simulink model "NN_Blackbox_comparison_Sinusoidal_24_24_6"  (R2019a)
settings: Solver=FixedStepAuto  StartTime=0.0  StopTime=10  FixedStep=0.01  RelTol=1e-3
undefined symbols (not defined in the file or in its folder): B, b, l, m, R
libraries: neural x17
(part 2 of 2)

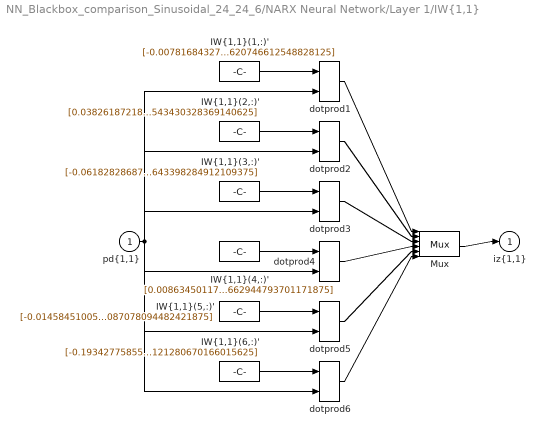
== system NN_Blackbox_comparison_Sinusoidal_24_24_6/NARX Neural Network/Layer 1/IW{1,1} ==
  "pd{1,1}" : Inport  PortDimensions=24  SampleTime=0.01
      mask Display: e = 0.06;c1 = [120 230 180]/255;c2 = ([120 230 180]+0)/(256+128);c3 = ([120 230 180]+128)/(256+128);patch([0 1 1 0],[0 0 1 1],c1);patch([0 1 1 1-e 1-e 0+e],[0 0 1 1-e 0+e 0+e],c2);patch([0 0 1 1-e 0+e 0+e],[0 1 1 1-e 1-e 0+e],c3);plot([0 1 1 0 0],[0 0 1 1 0]);
  "IW{1,1}(1,:)'" : Constant  Value=[-0.00781684327807324365322561021685032756067812442779541015625;-0.1850159880792916766711897480490733869373798370361328125;0.1001605115023758985071111737852334044873714447021484375;-0.1833831276225645068311820296003133989870548248291015625;-0.0494952264880428038917870026125456206500530242919921875;-0.0199884323316934509051634449861012399196624755859375;0.1165778684201735082570650092748110182583332061767578125;-0.1146125589407599176805518936816952191293239593505859375;0.05020117748370077348507578562930575571954250335693359375;-0.07054520144965477357335004171545733697712421417236328125;0.06259819221112832010600612875350634567439556121826171875;0.1424776467193929196941581949431565590202808380126953125;-0.133745237374407854868962886030203662812709808349609375;0.0296684098027802482799852867856316152028739452362060546875;0.00161749987780685660666846192867751597077585756778717041015625;-0.082135310527604088459696640711626969277858734130859375;0.017117640879136607201527198185431188903748989105224609375;-0.06257214896964193029393896949841291643679141998291015625;0.044772057090533036449730985850692377425730228424072265625;0.077435295268282799963088791628251783549785614013671875;0.05627579238971676389713394428326864726841449737548828125;-0.021855753086099154181010106867688591592013835906982421875;-0.1460877193397679130182353901545866392552852630615234375;-0.03835883480631437081331824856533785350620746612548828125]
      mask Display: e = 0.06;c1 = [120 150 230]/255;c2 = ([120 150 230]+0)/383;c3 = ([120 150 230]+128)/383;patch([0 1 1 0],[0 0 1 1],c1);patch([0 1 1 1-e 1-e 0+e],[0 0 1 1-e 0+e 0+e],c2);patch([0 0 1 1-e 0+e 0+e],[0 1 1 1-e 1-e 0+e],c3);plot([0 1 1 0 0],[0 0 1 1 0]);disp('Weights');
  "IW{1,1}(2,:)'" : Constant  Value=[0.0382618721846479659109974136299570091068744659423828125;-0.11423689285097904377863642366719432175159454345703125;0.133546945696815633208842655221815221011638641357421875;0.1881509242216309052420086800339049659669399261474609375;-0.310690738266952648505281331381411291658878326416015625;0.08079194265866813939869217620071140117943286895751953125;-0.1261531193252228566503703177659190259873867034912109375;0.22552293164817882598072174005210399627685546875;-0.262279279918452068454115533313597552478313446044921875;0.07233767871772382729300687742579611949622631072998046875;-0.0205932665107694153061590469633301836438477039337158203125;-0.1546453563928802121818506520867231301963329315185546875;0.036264331257236916139508053902318351902067661285400390625;0.04911111148654201397079077651142142713069915771484375;-0.13793151140202575266613393978332169353961944580078125;-0.07579443180956568770767489695572294294834136962890625;0.09929461869162765907947942878308822400867938995361328125;0.132426095028207180259727238080813549458980560302734375;-0.221957074010017019194407339455210603773593902587890625;-0.348947713802484626999245165279717184603214263916015625;-0.06397706287970154892530416645968216471374034881591796875;-0.08647843787593545439307263222872279584407806396484375;0.17868669570401685131599833766813389956951141357421875;0.1398750507253951058661556317019858397543430328369140625]
      mask Display: e = 0.06;c1 = [120 150 230]/255;c2 = ([120 150 230]+0)/383;c3 = ([120 150 230]+128)/383;patch([0 1 1 0],[0 0 1 1],c1);patch([0 1 1 1-e 1-e 0+e],[0 0 1 1-e 0+e 0+e],c2);patch([0 0 1 1-e 0+e 0+e],[0 1 1 1-e 1-e 0+e],c3);plot([0 1 1 0 0],[0 0 1 1 0]);disp('Weights');
  "IW{1,1}(3,:)'" : Constant  Value=[-0.061828286876414721706662902533935266546905040740966796875;-0.188069077398500261733005345377023331820964813232421875;-0.05601321185507872335573864575053448788821697235107421875;-0.855195451738412604214545353897847235202789306640625;-0.02152969126247221420822341997336479835212230682373046875;-0.1226276060420865288147496130477520637214183807373046875;0.54597989168019134265108505132957361638545989990234375;-0.472796354773704685658941571091418154537677764892578125;-0.05967068096914411590159232900987262837588787078857421875;0.07449502355572552858564705502431024797260761260986328125;0.432613897270532843375434595145634375512599945068359375;0.62244785617741282823800474943709559738636016845703125;-0.40187421715495552643204746345872990787029266357421875;0.11617911031940737764944771015507285483181476593017578125;-0.027881334145780554967242181874098605476319789886474609375;-0.2104685385077245118878863650024868547916412353515625;-0.0772998380072060786716292568598873913288116455078125;-0.37592925407182342656398077451740391552448272705078125;0.41876994636821718298591576967737637460231781005859375;0.63252910097631287467123684109537862241268157958984375;-0.07433228516414784603494325665451469831168651580810546875;0.01353334729246670649349670867422901210375130176544189453125;-0.62092193287436103776855134128709323704242706298828125;-0.486445315902774344518633142797625623643398284912109375]
      mask Display: e = 0.06;c1 = [120 150 230]/255;c2 = ([120 150 230]+0)/383;c3 = ([120 150 230]+128)/383;patch([0 1 1 0],[0 0 1 1],c1);patch([0 1 1 1-e 1-e 0+e],[0 0 1 1-e 0+e 0+e],c2);patch([0 0 1 1-e 0+e 0+e],[0 1 1 1-e 1-e 0+e],c3);plot([0 1 1 0 0],[0 0 1 1 0]);disp('Weights');
  "IW{1,1}(4,:)'" : Constant  Value=[0.00863450117239293428450519485295444610528647899627685546875;-0.000724270040755028749086819050972962941159494221210479736328125;0.0037910992940890044823609716928558555082418024539947509765625;0.00121298856381454205934089518592600143165327608585357666015625;0.0021858889202538661460095692490313012967817485332489013671875;0.0015493290437253895257263547335924158687703311443328857421875;0.00138676077665267328230258581100997616886161267757415771484375;0.00116498878916462887504745804534422859433107078075408935546875;0.000675385155924593358518770447318502192501910030841827392578125;0.000216059403336755378489952850173949627787806093692779541015625;0.000561817516077093973871081633575386149459518492221832275390625;0.000502256192877557319960424297988765829359181225299835205078125;0.0004713245037647317684827152906024139156215824186801910400390625;0.000252772431095591256812460390079877470270730555057525634765625;-9.378217509820683931744123018603431773954071104526519775390625e-05;-9.917273133467054894822634292239627029630355536937713623046875e-05;0.00022807121218579545600391167425868843565694987773895263671875;6.01539461235079875507138214008051591008552350103855133056640625e-05;0.00050922601514351360611765340280499003711156547069549560546875;-0.0003978415441667664041551499831683713637175969779491424560546875;0.00048009319238550250685815257156718871556222438812255859375;-0.0003596580952784336391268860122494288589223287999629974365234375;-7.3598210936802051468190455363327373561332933604717254638671875e-05;-0.00022865933921139785611580108604101724267820827662944793701171875]
      mask Display: e = 0.06;c1 = [120 150 230]/255;c2 = ([120 150 230]+0)/383;c3 = ([120 150 230]+128)/383;patch([0 1 1 0],[0 0 1 1],c1);patch([0 1 1 1-e 1-e 0+e],[0 0 1 1-e 0+e 0+e],c2);patch([0 0 1 1-e 0+e 0+e],[0 1 1 1-e 1-e 0+e],c3);plot([0 1 1 0 0],[0 0 1 1 0]);disp('Weights');
  "IW{1,1}(5,:)'" : Constant  Value=[-0.01458451005635619072975384113988184253685176372528076171875;-6.42425160279898690464384092280170079902745783329010009765625e-05;0.000617139824523241513516691458818286264431662857532501220703125;-0.0004628604352088678554853762303622488616383634507656097412109375;0.0002626759407408229434789659340054868152947165071964263916015625;0.00010283267385660473298460149127464546836563386023044586181640625;-0.00075071973850503507207088116359727791859768331050872802734375;0.0007176821664602243792951963285986494156531989574432373046875;-0.001986327739272509933232679912862295168451964855194091796875;-0.001627764366681831893768350738582739722914993762969970703125;-0.0004169956863333358957311725045968842096044681966304779052734375;-0.0018908506049463806586441450008351239375770092010498046875;9.8008331296605655474744878130621827949653379619121551513671875e-05;-0.0013958936559834863276596816916708121425472199916839599609375;-0.0022485379598983609890361368144340303842909634113311767578125;-0.00108820154986972463494188101407189606106840074062347412109375;-0.00049658626834902315667907846119533132878132164478302001953125;-0.0009511741998911474142708311063643122906796634197235107421875;0.0003314857832199900725990426852973769200616516172885894775390625;-0.003139569163090162075280264986076872446574270725250244140625;-0.00017847932028995896667177001315707229878171347081661224365234375;-0.002218879578591786451424727744097253889776766300201416015625;-0.000318328681633440655450451028940506148501299321651458740234375;-0.00113966174305159153971878094324665653402917087078094482421875]
      mask Display: e = 0.06;c1 = [120 150 230]/255;c2 = ([120 150 230]+0)/383;c3 = ([120 150 230]+128)/383;patch([0 1 1 0],[0 0 1 1],c1);patch([0 1 1 1-e 1-e 0+e],[0 0 1 1-e 0+e 0+e],c2);patch([0 0 1 1-e 0+e 0+e],[0 1 1 1-e 1-e 0+e],c3);plot([0 1 1 0 0],[0 0 1 1 0]);disp('Weights');
  "IW{1,1}(6,:)'" : Constant  Value=[-0.19342775855704219534203502917080186307430267333984375;0.1533401124560897776927248514766688458621501922607421875;-0.465714971164614188747776779564446769654750823974609375;-0.2452381847837121764399626044905744493007659912109375;-0.437933644939707600318712366060935892164707183837890625;0.0224203308941918477703580947490991093218326568603515625;0.6222688006434211605011341816862113773822784423828125;0.54116406477055345458637702904525212943553924560546875;0.55228269096517623726327883559861220419406890869140625;-0.364776363386681234945996266105794347822666168212890625;0.5125049224945821269017187660210765898227691650390625;-0.3208727112808242853958518026047386229038238525390625;0.26590788638917650654747149019385688006877899169921875;-0.42450676756308725057209585429518483579158782958984375;0.06490358610860956500854257456012419424951076507568359375;0.0253195955065332427291746597575183841399848461151123046875;0.1263078999877178254518383937465841881930828094482421875;-0.41212086410198878194677263309131376445293426513671875;-0.0396676510640926738293643438737490214407444000244140625;0.374919128482076313702009429107420146465301513671875;-0.262882740181810070634327303196187131106853485107421875;-0.420155000962919966678299488194170407950878143310546875;-0.682896272804139670142831164412200450897216796875;-0.031254028514375566116800797544783563353121280670166015625]
      mask Display: e = 0.06;c1 = [120 150 230]/255;c2 = ([120 150 230]+0)/383;c3 = ([120 150 230]+128)/383;patch([0 1 1 0],[0 0 1 1],c1);patch([0 1 1 1-e 1-e 0+e],[0 0 1 1-e 0+e 0+e],c2);patch([0 0 1 1-e 0+e 0+e],[0 1 1 1-e 1-e 0+e],c3);plot([0 1 1 0 0],[0 0 1 1 0]);disp('Weights');
  Mux : Mux  Inputs=6
      mask Display: e = 0.06;c1 = [120 150 230]/255;c2 = ([120 150 230]+0)/383;c3 = ([120 150 230]+128)/383;patch([0 1 1 0],[0 0 1 1],c1);patch([0 1 1 1-e 1-e 0+e],[0 0 1 1-e 0+e 0+e],c2);patch([0 0 1 1-e 0+e 0+e],[0 1 1 1-e 1-e 0+e],c3);plot([0 1 1 0 0],[0 0 1 1 0]);disp('Mux');
  dotprod{1..6} (6 alike) : neural/Weight Functions/dotprod
      settings: SourceProductName=MATLAB Runtime - Deep Learning Toolbox  SourceProductBaseCode=Missing
  "iz{1,1}" : Outport
      mask Display: e = 0.06;c1 = [120 230 180]/255;c2 = ([120 230 180]+0)/(256+128);c3 = ([120 230 180]+128)/(256+128);patch([0 1 1 0],[0 0 1 1],c1);patch([0 1 1 1-e 1-e 0+e],[0 0 1 1-e 0+e 0+e],c2);patch([0 0 1 1-e 0+e 0+e],[0 1 1 1-e 1-e 0+e],c3);plot([0 1 1 0 0],[0 0 1 1 0]);
  wires:
  "IW{1,1}(1,:)'"/1 -> dotprod1/1
  "pd{1,1}"/1 -> dotprod1/2, dotprod2/2, dotprod3/2, dotprod4/2, dotprod5/2, dotprod6/2
  dotprod1/1 -> Mux/1
  "IW{1,1}(2,:)'"/1 -> dotprod2/1
  dotprod2/1 -> Mux/2
  "IW{1,1}(3,:)'"/1 -> dotprod3/1
  dotprod3/1 -> Mux/3
  "IW{1,1}(4,:)'"/1 -> dotprod4/1
  dotprod4/1 -> Mux/4
  "IW{1,1}(5,:)'"/1 -> dotprod5/1
  dotprod5/1 -> Mux/5
  "IW{1,1}(6,:)'"/1 -> dotprod6/1
  dotprod6/1 -> Mux/6
  Mux/1 -> "iz{1,1}"/1

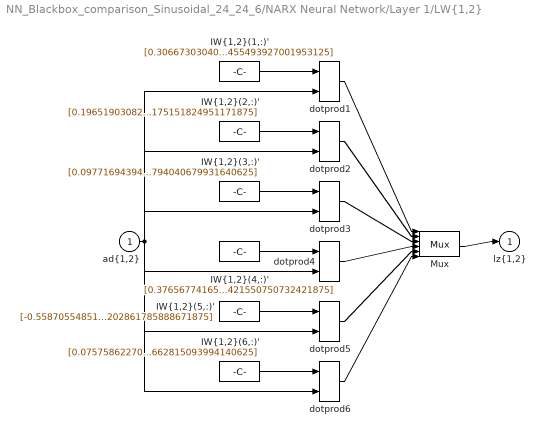
== system NN_Blackbox_comparison_Sinusoidal_24_24_6/NARX Neural Network/Layer 1/LW{1,2} ==
  "ad{1,2}" : Inport  PortDimensions=24  SampleTime=0.01
      mask Display: e = 0.06;c1 = [120 230 180]/255;c2 = ([120 230 180]+0)/(256+128);c3 = ([120 230 180]+128)/(256+128);patch([0 1 1 0],[0 0 1 1],c1);patch([0 1 1 1-e 1-e 0+e],[0 0 1 1-e 0+e 0+e],c2);patch([0 0 1 1-e 0+e 0+e],[0 1 1 1-e 1-e 0+e],c3);plot([0 1 1 0 0],[0 0 1 1 0]);
  "IW{1,2}(1,:)'" : Constant  Value=[0.306673030408703917171209241132601164281368255615234375;-0.11198177206757127521985495377521147020161151885986328125;0.3269859355907691611520249352906830608844757080078125;0.056270185849424024515652575928470469079911708831787109375;-0.113558622384051233211721410043537616729736328125;0.09782792362847221590005375446708058007061481475830078125;-0.3122359510233196910888864294975064694881439208984375;-0.257081540505827488285461868144921027123928070068359375;0.276391847125739553714396379291429184377193450927734375;0.2222602218884729696757318606614717282354831695556640625;-0.2021395968177663593490223092885571531951427459716796875;0.1814053757736827365842913195592700503766536712646484375;0.2258593327786559690206757977648521773517131805419921875;-0.2029117090672250822702693540122709237039089202880859375;0.0282557608137135353454372221904122852720320224761962890625;-0.230249871903323855004686038228101097047328948974609375;-0.2195438158585874266481852146171149797737598419189453125;0.261170925858878799630247158347629010677337646484375;0.180486427927954939942623013848788104951381683349609375;0.069226347620993278209056143168709240853786468505859375;-0.1443199707426636724250101906363852322101593017578125;-0.2391833789258829556789720527376630343496799468994140625;0.1659067472852251701187498156286892481148242950439453125;0.11194979810412608589587080132332630455493927001953125]
      mask Display: e = 0.06;c1 = [120 150 230]/255;c2 = ([120 150 230]+0)/383;c3 = ([120 150 230]+128)/383;patch([0 1 1 0],[0 0 1 1],c1);patch([0 1 1 1-e 1-e 0+e],[0 0 1 1-e 0+e 0+e],c2);patch([0 0 1 1-e 0+e 0+e],[0 1 1 1-e 1-e 0+e],c3);plot([0 1 1 0 0],[0 0 1 1 0]);disp('weights');
  "IW{1,2}(2,:)'" : Constant  Value=[0.196519030828230689689206656112219206988811492919921875;-0.1595862747555963634393805250510922633111476898193359375;-0.238312071756647425591069122674525715410709381103515625;-0.37667022763899893345040936765144579112529754638671875;-0.01219480248024964845476869612639347906224429607391357421875;-0.16186153809693315519524503542925231158733367919921875;-0.10963349883229563108688608963348087854683399200439453125;0.08577468354507998549163261259309365414083003997802734375;-0.13244028970139598566646554900216870009899139404296875;0.06973027897582433076717478570571984164416790008544921875;0.1996874709654370416700430723722092807292938232421875;0.1414539201875719409695619788180920295417308807373046875;-0.410338678032958481534109296262613497674465179443359375;0.2175943984202941272609876932619954459369182586669921875;0.1394821677224036549080921076892991550266742706298828125;0.0428180467314927259980805729355779476463794708251953125;-0.275353647726182426680452408618293702602386474609375;0.05862862738383915750528529997609439305961132049560546875;0.13762278415745765602906658386928029358386993408203125;-0.136380748418356068096812805379158817231655120849609375;-0.393208750383996219479598721591173671185970306396484375;-0.41983179452645702500745983343222178518772125244140625;0.0193259477496929565898398095669108442962169647216796875;0.051822453742941747278916153618411044590175151824951171875]
      mask Display: e = 0.06;c1 = [120 150 230]/255;c2 = ([120 150 230]+0)/383;c3 = ([120 150 230]+128)/383;patch([0 1 1 0],[0 0 1 1],c1);patch([0 1 1 1-e 1-e 0+e],[0 0 1 1-e 0+e 0+e],c2);patch([0 0 1 1-e 0+e 0+e],[0 1 1 1-e 1-e 0+e],c3);plot([0 1 1 0 0],[0 0 1 1 0]);disp('weights');
  "IW{1,2}(3,:)'" : Constant  Value=[0.09771694394740902678275773496352485381066799163818359375;-0.1415025473628825636307482227493892423808574676513671875;0.1755285439126030022638502714471542276442050933837890625;0.1116232255050156052522680738547933287918567657470703125;-0.34408022982841279802102008034125901758670806884765625;0.0792148754280949385364607451265328563749790191650390625;0.266739206129793571253827622058452107012271881103515625;0.2537797995477009127540668487199582159519195556640625;0.305212184974735178943916480420739389955997467041015625;-0.3149703916652015767141392643679864704608917236328125;0.264525796061264750758112995754345320165157318115234375;-0.2530632579431484341370151014416478574275970458984375;0.025395663220353130451467649209007504396140575408935546875;0.2409238223387252519902546055163838900625705718994140625;0.32858810067802923793323088830220513045787811279296875;-0.261318748295446268148367607864202000200748443603515625;0.1881791957386545754982165590263321064412593841552734375;-0.10850413491654682662801434389621135778725147247314453125;0.2217647526361911924919212424356373958289623260498046875;-0.31005730369838302440399502302170731127262115478515625;0.05467111885891319522645659390036598779261112213134765625;0.210146756312323101933969837773474864661693572998046875;0.341591394286220928488972958803060464560985565185546875;0.17273883000019341071862299941130913794040679931640625]
      mask Display: e = 0.06;c1 = [120 150 230]/255;c2 = ([120 150 230]+0)/383;c3 = ([120 150 230]+128)/383;patch([0 1 1 0],[0 0 1 1],c1);patch([0 1 1 1-e 1-e 0+e],[0 0 1 1-e 0+e 0+e],c2);patch([0 0 1 1-e 0+e 0+e],[0 1 1 1-e 1-e 0+e],c3);plot([0 1 1 0 0],[0 0 1 1 0]);disp('weights');
  "IW{1,2}(4,:)'" : Constant  Value=[0.376567741656371468561559368026792071759700775146484375;-0.226796412015716819521315983365639112889766693115234375;0.1288925676318834756539644104122999124228954315185546875;-0.0703574015836986033090028058722964487969875335693359375;0.036116553042721107058543594803268206305801868438720703125;0.00456047255372171549125948075698033790104091167449951171875;-0.003630385408504195610124298809751053340733051300048828125;0.016596451191842331862602577530196867883205413818359375;0.007788283319363454963724091584253983455710113048553466796875;-0.01299859135048583337612715382647365913726389408111572265625;0.01145889041297005160602306972350561409257352352142333984375;-0.01316943770400048896451750124469981528818607330322265625;0.018599606798864846968211139710547286085784435272216796875;0.0029078928036930192825570973269577734754420816898345947265625;-0.00020205609617424431377792626296496791837853379547595977783203125;-0.007535644507239321054914427122639608569443225860595703125;0.00942303876382953424506450090802900376729667186737060546875;-0.0306685189480544635742820247514828224666416645050048828125;0.0431527151917643070344610123356687836349010467529296875;-0.03292662848017215149187819633880280889570713043212890625;0.0289622948350503235659392231582387466914951801300048828125;-0.0157427143958187194805464770297476206906139850616455078125;0.01559357247640663461651922006012682686559855937957763671875;-0.0123741206487570643002271708610351197421550750732421875]
      mask Display: e = 0.06;c1 = [120 150 230]/255;c2 = ([120 150 230]+0)/383;c3 = ([120 150 230]+128)/383;patch([0 1 1 0],[0 0 1 1],c1);patch([0 1 1 1-e 1-e 0+e],[0 0 1 1-e 0+e 0+e],c2);patch([0 0 1 1-e 0+e 0+e],[0 1 1 1-e 1-e 0+e],c3);plot([0 1 1 0 0],[0 0 1 1 0]);disp('weights');
  "IW{1,2}(5,:)'" : Constant  Value=[-0.55870554851228948489705317115294747054576873779296875;0.07272659225011755823597781045464216731488704681396484375;0.054468456770181673809450018097777501679956912994384765625;-0.08931506060536253954751373385079205036163330078125;0.03757319402559498866533971295211813412606716156005859375;0.033882810130841621576447408870080835185945034027099609375;-0.0316717851875283062934585132097708992660045623779296875;0.034115471430612130665505077331545180641114711761474609375;0.039509450488714951965629751384767587296664714813232421875;-0.08457828136277301123158167683868668973445892333984375;0.0684207651316723064471858606339083053171634674072265625;-0.05757860294501955522594727199248154647648334503173828125;0.05457062570232155962468567622636328451335430145263671875;0.00171703879725057842985103118138567879213951528072357177734375;-0.0104754842807108887459133228503560530953109264373779296875;-0.022728858084237961445506215341083589009940624237060546875;0.046300541575451915898842258911827229894697666168212890625;-0.11998735138502857056064243579385220073163509368896484375;0.16380339683133848804885701611055992543697357177734375;-0.1380869937040725137222807461512275040149688720703125;0.113004389650570191694356481093564070761203765869140625;-0.0573476784986787502251814885312342084944248199462890625;0.035521598388957374703434055618345155380666255950927734375;-0.049287448855453823426397974571955273859202861785888671875]
      mask Display: e = 0.06;c1 = [120 150 230]/255;c2 = ([120 150 230]+0)/383;c3 = ([120 150 230]+128)/383;patch([0 1 1 0],[0 0 1 1],c1);patch([0 1 1 1-e 1-e 0+e],[0 0 1 1-e 0+e 0+e],c2);patch([0 0 1 1-e 0+e 0+e],[0 1 1 1-e 1-e 0+e],c3);plot([0 1 1 0 0],[0 0 1 1 0]);disp('weights');
  "IW{1,2}(6,:)'" : Constant  Value=[0.0757586227050215388345577594009228050708770751953125;-0.27684473270092035956935205831541679799556732177734375;0.264526169646414455183247582681360654532909393310546875;-0.2888354913074187013677374125109054148197174072265625;-0.3042240724428435516557556184125132858753204345703125;0.2296829497905580608207998238867730833590030670166015625;0.09251050887686319834646297977087670005857944488525390625;0.37829873239017264285877217844245024025440216064453125;0.06326772721295646773054244249578914605081081390380859375;0.19124998334157528034893402946181595325469970703125;0.04753677910932539718569245223989128135144710540771484375;0.015009511298633780584932395640862523578107357025146484375;0.07473145941779786582959133056647260673344135284423828125;0.2185796547470139350455298199449316598474979400634765625;0.335696523217766384927784883984713815152645111083984375;-0.1889761753167945868003840814708382822573184967041015625;-0.2552293769360109987331952652311883866786956787109375;0.169419213418987746333499444517656229436397552490234375;-0.03779132130635280695241107196125085465610027313232421875;0.0046226941957490420842535883139134966768324375152587890625;-0.031016369668211217491826658942954964004456996917724609375;-0.319486968289223849382096886984072625637054443359375;0.2340934549271946607529315542706171981990337371826171875;-0.33456530111625470969016760136582888662815093994140625]
      mask Display: e = 0.06;c1 = [120 150 230]/255;c2 = ([120 150 230]+0)/383;c3 = ([120 150 230]+128)/383;patch([0 1 1 0],[0 0 1 1],c1);patch([0 1 1 1-e 1-e 0+e],[0 0 1 1-e 0+e 0+e],c2);patch([0 0 1 1-e 0+e 0+e],[0 1 1 1-e 1-e 0+e],c3);plot([0 1 1 0 0],[0 0 1 1 0]);disp('weights');
  Mux : Mux  Inputs=6
      mask Display: e = 0.06;c1 = [120 150 230]/255;c2 = ([120 150 230]+0)/383;c3 = ([120 150 230]+128)/383;patch([0 1 1 0],[0 0 1 1],c1);patch([0 1 1 1-e 1-e 0+e],[0 0 1 1-e 0+e 0+e],c2);patch([0 0 1 1-e 0+e 0+e],[0 1 1 1-e 1-e 0+e],c3);plot([0 1 1 0 0],[0 0 1 1 0]);disp('Mux');
  dotprod{1..6} (6 alike) : neural/Weight Functions/dotprod
      settings: SourceProductName=MATLAB Runtime - Deep Learning Toolbox  SourceProductBaseCode=Missing
  "lz{1,2}" : Outport
      mask Display: e = 0.06;c1 = [120 230 180]/255;c2 = ([120 230 180]+0)/(256+128);c3 = ([120 230 180]+128)/(256+128);patch([0 1 1 0],[0 0 1 1],c1);patch([0 1 1 1-e 1-e 0+e],[0 0 1 1-e 0+e 0+e],c2);patch([0 0 1 1-e 0+e 0+e],[0 1 1 1-e 1-e 0+e],c3);plot([0 1 1 0 0],[0 0 1 1 0]);
  wires:
  "IW{1,2}(1,:)'"/1 -> dotprod1/1
  "ad{1,2}"/1 -> dotprod1/2, dotprod2/2, dotprod3/2, dotprod4/2, dotprod5/2, dotprod6/2
  dotprod1/1 -> Mux/1
  "IW{1,2}(2,:)'"/1 -> dotprod2/1
  dotprod2/1 -> Mux/2
  "IW{1,2}(3,:)'"/1 -> dotprod3/1
  dotprod3/1 -> Mux/3
  "IW{1,2}(4,:)'"/1 -> dotprod4/1
  dotprod4/1 -> Mux/4
  "IW{1,2}(5,:)'"/1 -> dotprod5/1
  dotprod5/1 -> Mux/5
  "IW{1,2}(6,:)'"/1 -> dotprod6/1
  dotprod6/1 -> Mux/6
  Mux/1 -> "lz{1,2}"/1

== system NN_Blackbox_comparison_Sinusoidal_24_24_6/NARX Neural Network/Layer 2/Delays 1 ==
  "p{2}" : Inport  PortDimensions=6  SampleTime=0.01
      mask Display: e = 0.06;c1 = [120 230 180]/255;c2 = ([120 230 180]+0)/(256+128);c3 = ([120 230 180]+128)/(256+128);patch([0 1 1 0],[0 0 1 1],c1);patch([0 1 1 1-e 1-e 0+e],[0 0 1 1-e 0+e 0+e],c2);patch([0 0 1 1-e 0+e 0+e],[0 1 1 1-e 1-e 0+e],c3);plot([0 1 1 0 0],[0 0 1 1 0]);
  mux : Mux  Inputs=1
      mask Display: e = 0.06;c1 = [120 150 230]/255;c2 = ([120 150 230]+0)/383;c3 = ([120 150 230]+128)/383;patch([0 1 1 0],[0 0 1 1],c1);patch([0 1 1 1-e 1-e 0+e],[0 0 1 1-e 0+e 0+e],c2);patch([0 0 1 1-e 0+e 0+e],[0 1 1 1-e 1-e 0+e],c3);plot([0 1 1 0 0],[0 0 1 1 0]);disp('Mux')
  "pd{2,1}" : Outport
      mask Display: e = 0.06;c1 = [120 230 180]/255;c2 = ([120 230 180]+0)/(256+128);c3 = ([120 230 180]+128)/(256+128);patch([0 1 1 0],[0 0 1 1],c1);patch([0 1 1 1-e 1-e 0+e],[0 0 1 1-e 0+e 0+e],c2);patch([0 0 1 1-e 0+e 0+e],[0 1 1 1-e 1-e 0+e],c3);plot([0 1 1 0 0],[0 0 1 1 0]);
  wires:
  "p{2}"/1 -> mux/1
  mux/1 -> "pd{2,1}"/1

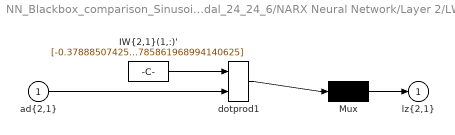
== system NN_Blackbox_comparison_Sinusoidal_24_24_6/NARX Neural Network/Layer 2/LW{2,1} ==
  "ad{2,1}" : Inport  PortDimensions=6  SampleTime=0.01
      mask Display: e = 0.06;c1 = [120 230 180]/255;c2 = ([120 230 180]+0)/(256+128);c3 = ([120 230 180]+128)/(256+128);patch([0 1 1 0],[0 0 1 1],c1);patch([0 1 1 1-e 1-e 0+e],[0 0 1 1-e 0+e 0+e],c2);patch([0 0 1 1-e 0+e 0+e],[0 1 1 1-e 1-e 0+e],c3);plot([0 1 1 0 0],[0 0 1 1 0]);
  "IW{2,1}(1,:)'" : Constant  Value=[-0.378885074258745568887007948433165438473224639892578125;0.002013940415117906716779838660613677348010241985321044921875;0.001397711243469999635447020835954390349797904491424560546875;3.04057341128410474340171276708133518695831298828125;-1.10259388683669801167752666515298187732696533203125;0.000710811807877522795241775899199865307309664785861968994140625]
      mask Display: e = 0.06;c1 = [120 150 230]/255;c2 = ([120 150 230]+0)/383;c3 = ([120 150 230]+128)/383;patch([0 1 1 0],[0 0 1 1],c1);patch([0 1 1 1-e 1-e 0+e],[0 0 1 1-e 0+e 0+e],c2);patch([0 0 1 1-e 0+e 0+e],[0 1 1 1-e 1-e 0+e],c3);plot([0 1 1 0 0],[0 0 1 1 0]);disp('weights');
  Mux : Mux  Inputs=1
      mask Display: e = 0.06;c1 = [120 150 230]/255;c2 = ([120 150 230]+0)/383;c3 = ([120 150 230]+128)/383;patch([0 1 1 0],[0 0 1 1],c1);patch([0 1 1 1-e 1-e 0+e],[0 0 1 1-e 0+e 0+e],c2);patch([0 0 1 1-e 0+e 0+e],[0 1 1 1-e 1-e 0+e],c3);plot([0 1 1 0 0],[0 0 1 1 0]);disp('Mux');
  dotprod1 : neural/Weight Functions/dotprod
      settings: SourceProductName=MATLAB Runtime - Deep Learning Toolbox  SourceProductBaseCode=Missing
  "lz{2,1}" : Outport
      mask Display: e = 0.06;c1 = [120 230 180]/255;c2 = ([120 230 180]+0)/(256+128);c3 = ([120 230 180]+128)/(256+128);patch([0 1 1 0],[0 0 1 1],c1);patch([0 1 1 1-e 1-e 0+e],[0 0 1 1-e 0+e 0+e],c2);patch([0 0 1 1-e 0+e 0+e],[0 1 1 1-e 1-e 0+e],c3);plot([0 1 1 0 0],[0 0 1 1 0]);
  wires:
  "IW{2,1}(1,:)'"/1 -> dotprod1/1
  "ad{2,1}"/1 -> dotprod1/2
  dotprod1/1 -> Mux/1
  Mux/1 -> "lz{2,1}"/1
